simulink model "F1_Telemetry_Simple"  (R2025a)
settings: Solver=FixedStepAuto  StartTime=0.0  StopTime=30  FixedStep=0.1  RelTol=1e-3
settings Model: Creator=sunda  LastModifiedBy=sunda

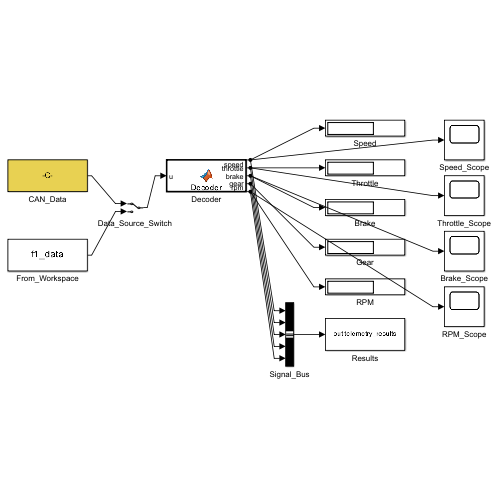
[thumbnail: Simulink's stored preview of the top-level diagram]
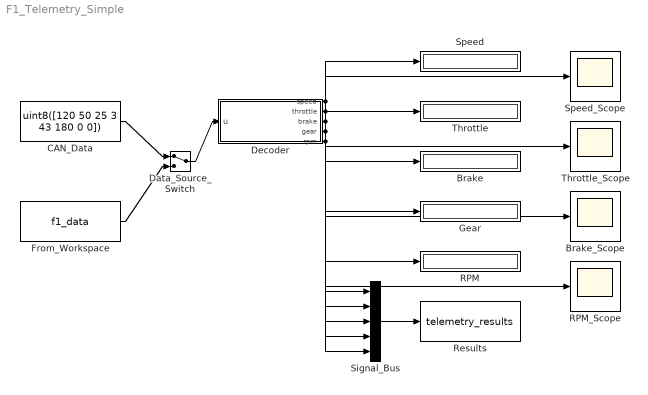
== system F1_Telemetry_Simple ==
  Brake : Display
  Brake_Scope : Scope
  CAN_Data : Constant  Value=uint8([120 50 25 3 43 180 0 0])  OutDataTypeStr=uint8
  Data_Source_Switch : ManualSwitch
  Decoder : MATLAB Function  TreatAsAtomicUnit=on
  From_Workspace : FromWorkspace  VariableName=f1_data
  Gear : Display
  RPM : Display
  RPM_Scope : Scope
  Results : ToWorkspace  VariableName=telemetry_results  SaveFormat=Timeseries  SampleTime=-1
  Signal_Bus : BusCreator  Inputs=5
  Speed : Display
  Speed_Scope : Scope
  Throttle : Display
  Throttle_Scope : Scope
  wires:
  CAN_Data/1 -> Data_Source_Switch/1
  Decoder/1(speed) -> Speed/1, Speed_Scope/1, Signal_Bus/1
  Decoder/2(throttle) -> Throttle/1, Throttle_Scope/1, Signal_Bus/2
  Decoder/3(brake) -> Brake/1, Brake_Scope/1, Signal_Bus/3
  Decoder/4(gear) -> Gear/1, Signal_Bus/4
  Decoder/5(rpm) -> RPM/1, RPM_Scope/1, Signal_Bus/5
  From_Workspace/1 -> Data_Source_Switch/2
  Data_Source_Switch/1 -> Decoder/1(u)
  Signal_Bus/1 -> Results/1

== matlab function F1_Telemetry_Simple/Decoder ==
  data: u input; speed output; throttle output; brake output; gear output; rpm output
function [speed, throttle, brake, gear, rpm] = Decoder(u)
    speed = double(u(1));
    throttle = double(u(2));
    brake = double(u(3));
    gear = double(u(4));
    rpm = double(bitshift(u(5), 8) + u(6));
end
